simulink model "Control"  (Simulink 9.1)
settings: Solver=ode45  StartTime=0.0  StopTime=4  MaxStep=1e-3  RelTol=1e-3  EnableMultiTasking=on
undefined symbols (not defined in the file): CinematicaDirecta, Kd, Ki, Kp, Tm
settings Model: Creator=mortega  LastModifiedBy=rafap  ExtModeTrigMode=oneshot  ExtModeArmWhenConnect=off
settings DataIOCC: SignalLoggingSaveFormat=ModelDataLogs
settings OptimizationCC: BlockReduction=off  BooleanDataType=off  ExpressionDepthLimit=2147483647  InitFltsAndDblsToZero=on
settings DebuggingCC: SaveWithParameterizedLinksMsg=none  SignalResolutionControl=TryResolveAllWithWarning  MultiTaskDSMMsg=warning  MultiTaskCondExecSysMsg=none  FcnCallInpInsideContextMsg=warning  StateNameClashWarn=warning
settings HardwareCC: TargetUnknown=on
settings GRTTargetCC: TargetFcnLib=ansi_tfl_tmw.mat  GeneratePreprocessorConditionals=Disable all
settings ConfigComp: CovSFcnEnable=off

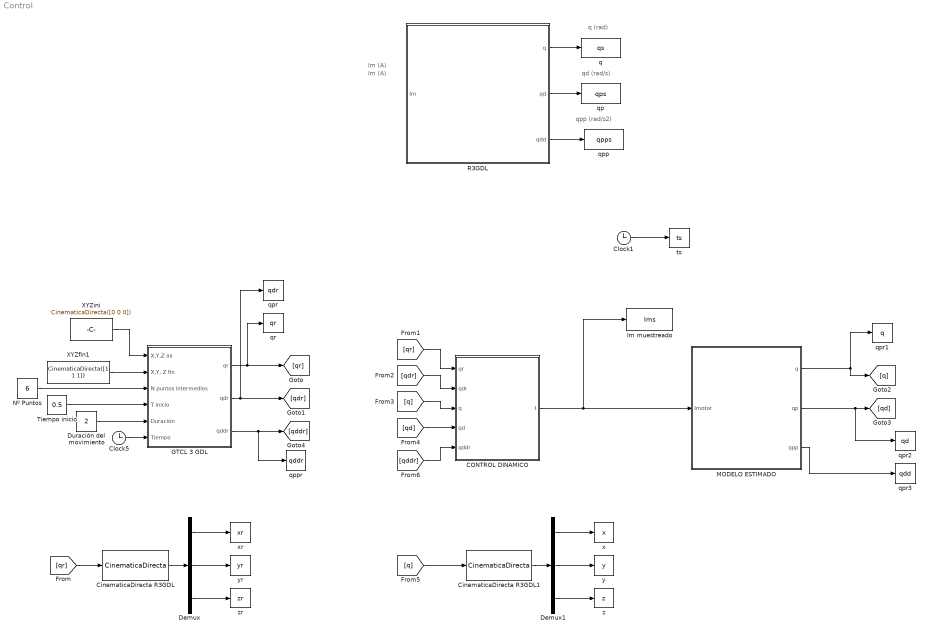
== system Control ==
  note: Im (A)
  note: q (rad)
  note: qd (rad/s)
  note: qpp (rad/s2)
  note: Im (A)
  CONTROL DINAMICO : Subsystem
  CinematicaDirecta R3GDL : MATLABFcn  MATLABFcn=CinematicaDirecta
  CinematicaDirecta R3GDL1 : MATLABFcn  MATLABFcn=CinematicaDirecta
  Clock1 : Clock
  Clock5 : Clock
  Demux : Demux  Outputs=3
  Demux1 : Demux  Outputs=3
  Duración del movimiento : Constant  Value=2
  GTCL 3 GDL : Subsystem
  Im muestreado : ToWorkspace  VariableName=Ims  SampleTime=Tm
  MODELO ESTIMADO : Subsystem
  Nº Puntos : Constant  Value=6
  R3GDL : Subsystem  mask(Control y Programación de Robots (4 GIERM)){NGrupo=13, q1_ini=0, q2_ini=0, q3_ini=0, Bl_q1=off, Bl_q2=off, Bl_q3=off, AccionamientoDirecto=on}
      mask prompts: NGrupo "Nº de GRUPO"; q1_ini "q1 inicial  (rad)"; q2_ini "q2 inicial (rad)"; q3_ini "q3_inicial (rad)"; Bl_q1 "Bloqueo q1"; Bl_q2 "Bloqueo q2"; Bl_q3 "Bloqueo q3"; AccionamientoDirecto "Accionamiento directo"
      mask help: Robot de 3 grados de libertad RRR
      mask Display:
      | image(imread('R3GDL_RRR.JPG'));
      | port_label('output', 1, 'q');
      | port_label('output', 2, 'qd');
      | port_label('output', 3, 'qdd');
      | port_label('input', 1, 'Im')
  Tiempo inicio : Constant  Value=0.5
  XYZfin1 : Constant  Value=CinematicaDirecta([1 1 1])
  XYZini : Constant  Value=CinematicaDirecta([0 0 0])
  q : ToWorkspace  VariableName=qs  SampleTime=1e-3
  qp : ToWorkspace  VariableName=qps  SampleTime=1e-3
  qpp : ToWorkspace  VariableName=qpps  SampleTime=1e-3
  qppr : ToWorkspace  VariableName=qddr  SampleTime=Tm
  qpr : ToWorkspace  VariableName=qdr  SampleTime=Tm
  qpr1 : ToWorkspace  VariableName=q  SampleTime=Tm
  qpr2 : ToWorkspace  VariableName=qd  SampleTime=Tm
  qpr3 : ToWorkspace  VariableName=qdd  SampleTime=Tm
  qr : ToWorkspace  VariableName=qr  SampleTime=Tm
  ts : ToWorkspace  VariableName=ts  SampleTime=Tm
  x : ToWorkspace  VariableName=x  SampleTime=Tm
  xr : ToWorkspace  VariableName=xr  SampleTime=Tm
  y : ToWorkspace  VariableName=y  SampleTime=Tm
  yr : ToWorkspace  VariableName=yr  SampleTime=Tm
  z : ToWorkspace  VariableName=z  SampleTime=Tm
  zr : ToWorkspace  VariableName=zr  SampleTime=Tm
  wires:
  R3GDL/1(q) -> q/1
  R3GDL/2(qd) -> qp/1
  R3GDL/3(qdd) -> qpp/1
  Clock1/1 -> ts/1
  GTCL 3 GDL/2(qdr) -> [qdr], qpr/1
  Demux1/1 -> x/1
  Demux/3 -> zr/1
  [qdr] -> CONTROL DINAMICO/2(qdr)
  Demux1/3 -> z/1
  MODELO ESTIMADO/3(qpp) -> qpr3/1
  CONTROL DINAMICO/1(I) -> Im muestreado/1, MODELO ESTIMADO/1(Imotor)
  [qddr] -> CONTROL DINAMICO/5(qddr)
  [q] -> CinematicaDirecta R3GDL1/1
  MODELO ESTIMADO/1(q) -> [q], qpr1/1
  CinematicaDirecta R3GDL1/1 -> Demux1/1
  Demux/2 -> yr/1
  Clock5/1 -> GTCL 3 GDL/6(Tiempo)
  Demux1/2 -> y/1
  [q] -> CONTROL DINAMICO/3(q)
  [qd] -> CONTROL DINAMICO/4(qd)
  [qr] -> CinematicaDirecta R3GDL/1
  MODELO ESTIMADO/2(qp) -> qpr2/1, [qd]
  Nº Puntos/1 -> GTCL 3 GDL/3(N puntos intermedios)
  GTCL 3 GDL/1(qr) -> qr/1, [qr]
  XYZfin1/1 -> GTCL 3 GDL/2("X,Y, Z fin")
  Demux/1 -> xr/1
  XYZini/1 -> GTCL 3 GDL/1(X,Y,Z ini)
  GTCL 3 GDL/3(qddr) -> [qddr], qppr/1
  Tiempo inicio/1 -> GTCL 3 GDL/4(T inicio)
  [qr] -> CONTROL DINAMICO/1(qr)
  Duración del movimiento/1 -> GTCL 3 GDL/5(Duración)
  CinematicaDirecta R3GDL/1 -> Demux/1

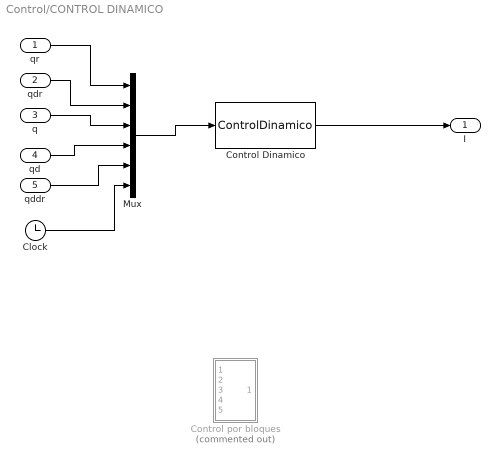
== system Control/CONTROL DINAMICO ==
  qr : Inport
  qdr : Inport  Port=2
  q : Inport  Port=3
  qd : Inport  Port=4
  qddr : Inport  Port=5
  Clock : Clock
  Control Dinamico : MATLABFcn  MATLABFcn=ControlDinamico
  Control por bloques : Subsystem  Commented=on
  Mux : Mux  Inputs=6
  I : Outport
  wires:
  Control Dinamico/1 -> I/1
  Mux/1 -> Control Dinamico/1
  qr/1 -> Mux/1
  qdr/1 -> Mux/2
  q/1 -> Mux/3
  qd/1 -> Mux/4
  qddr/1 -> Mux/5
  Clock/1 -> Mux/6

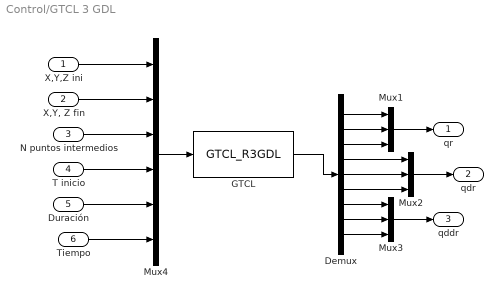
== system Control/GTCL 3 GDL ==
  X,Y,Z ini : Inport
  "X,Y, Z fin" : Inport  Port=2
  N puntos intermedios : Inport  Port=3
  T inicio : Inport  Port=4
  Duración : Inport  Port=5
  Tiempo : Inport  Port=6
  Demux : Demux  Outputs=9
  GTCL : MATLABFcn  MATLABFcn=GTCL_R3GDL  OutputDimensions=9
  Mux1 : Mux  Inputs=3
  Mux2 : Mux  Inputs=3
  Mux3 : Mux  Inputs=3
  Mux4 : Mux  Inputs=6
  qr : Outport
  qdr : Outport  Port=2
  qddr : Outport  Port=3
  wires:
  Mux1/1 -> qr/1
  Mux4/1 -> GTCL/1
  X,Y,Z ini/1 -> Mux4/1
  "X,Y, Z fin"/1 -> Mux4/2
  N puntos intermedios/1 -> Mux4/3
  T inicio/1 -> Mux4/4
  Duración/1 -> Mux4/5
  Tiempo/1 -> Mux4/6
  GTCL/1 -> Demux/1
  Demux/1 -> Mux1/1
  Demux/2 -> Mux1/2
  Demux/3 -> Mux1/3
  Mux2/1 -> qdr/1
  Demux/4 -> Mux2/1
  Demux/5 -> Mux2/2
  Demux/6 -> Mux2/3
  Mux3/1 -> qddr/1
  Demux/7 -> Mux3/1
  Demux/8 -> Mux3/2
  Demux/9 -> Mux3/3

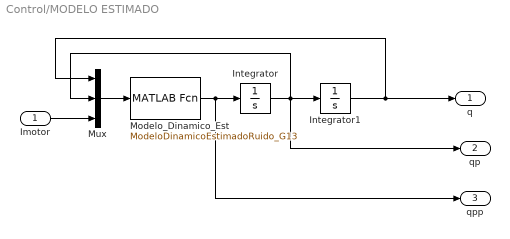
== system Control/MODELO ESTIMADO ==
  Imotor : Inport
  Integrator : Integrator  InitialCondition=[0;0;0]
  Integrator1 : Integrator  InitialCondition=[0;0;0]
  Modelo_Dinamico_Est : MATLABFcn  MATLABFcn=ModeloDinamicoEstimadoRuido_G13  OutputDimensions=3
  Mux : Mux  Inputs=3
  q : Outport
  qp : Outport  Port=2
  qpp : Outport  Port=3
  wires:
  Imotor/1 -> Mux/3
  Integrator1/1 -> Mux/1, q/1
  Integrator/1 -> Mux/2, qp/1, Integrator1/1
  Modelo_Dinamico_Est/1 -> qpp/1, Integrator/1
  Mux/1 -> Modelo_Dinamico_Est/1

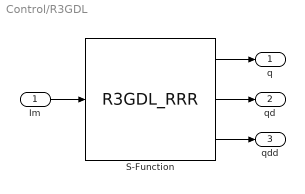
== system Control/R3GDL ==
  Im : Inport
  S-Function : S-Function  FunctionName=R3GDL_RRR  Parameters=[q1_ini; q2_ini; q3_ini]; [Bl_q1; Bl_q2; Bl_q3]; AccionamientoDirecto; NGrupo  SFunctionDeploymentMode=off  EnableBusSupport=off
  q : Outport
  qd : Outport  Port=2
  qdd : Outport  Port=3
  wires:
  Im/1 -> S-Function/1
  S-Function/1 -> q/1
  S-Function/2 -> qd/1
  S-Function/3 -> qdd/1

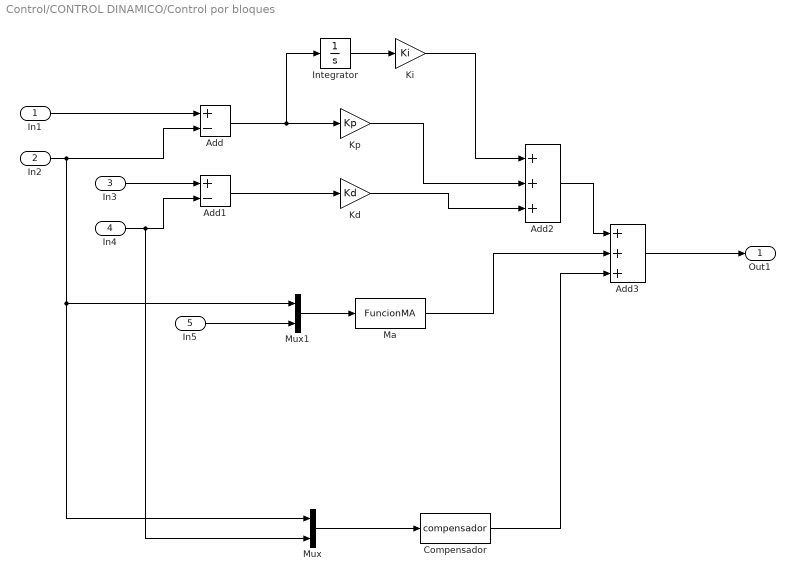
== system Control/CONTROL DINAMICO/Control por bloques ==
  In1 : Inport
  In2 : Inport  Port=2
  In3 : Inport  Port=3
  In4 : Inport  Port=4
  In5 : Inport  Port=5
  Add : Sum  Inputs=+-
  Add1 : Sum  Inputs=+-
  Add2 : Sum  Inputs=+++
  Add3 : Sum  Inputs=+++
  Compensador : MATLABFcn  MATLABFcn=compensador
  Integrator : Integrator
  Kd : Gain  Gain=Kd
  "Ki " : Gain  Gain=Ki
  "Kp " : Gain  Gain=Kp
  Ma : MATLABFcn  MATLABFcn=FuncionMA
  Mux : Mux  Inputs=2
  Mux1 : Mux  Inputs=2
  Out1 : Outport
  wires:
  In1/1 -> Add/1
  Mux1/1 -> Ma/1
  In3/1 -> Add1/1
  Add2/1 -> Add3/1
  Integrator/1 -> "Ki "/1
  "Kp "/1 -> Add2/2
  In2/1 -> Mux1/1, Mux/1, Add/2
  In4/1 -> Mux/2, Add1/2
  Add3/1 -> Out1/1
  In5/1 -> Mux1/2
  Compensador/1 -> Add3/3
  Mux/1 -> Compensador/1
  Add1/1 -> Kd/1
  Ma/1 -> Add3/2
  "Ki "/1 -> Add2/1
  Add/1 -> Integrator/1, "Kp "/1
  Kd/1 -> Add2/3
